simulink model "emg"  (R2014b)
settings: Solver=VariableStepAuto  StartTime=0.0  StopTime=10.0  RelTol=1e-3
libraries: simulink x1, instrumentlib x1, slrtlib x1
settings Model: Creator=Yue  LastModifiedBy=mLocal
settings DataIOCC: SaveFormat=Dataset
settings OptimizationCC: UseDivisionForNetSlopeComputation=off  SimCompilerOptimization=off
settings DebuggingCC: SolverPrmCheckMsg=none  FrameProcessingCompatibilityMsg=error  AllowSymbolicDim=off
settings HardwareCC: ProdBitPerPointer=64  ProdLargestAtomicFloat=Float  ProdIntDivRoundTo=Zero  ProdEndianess=LittleEndian  ProdHWDeviceType=Intel->x86-64 (Windows64)
settings RTWCC: RTWCompilerOptimization=off
settings GRTTargetCC: GeneratePreprocessorConditionals=Use local settings
settings ConfigComp: CovMetricSettings=dw  CovHtmlReporting=on  CovSaveCumulativeToWorkspaceVar=on  CovSaveSingleToWorkspaceVar=on  CovExternalEMLEnable=off

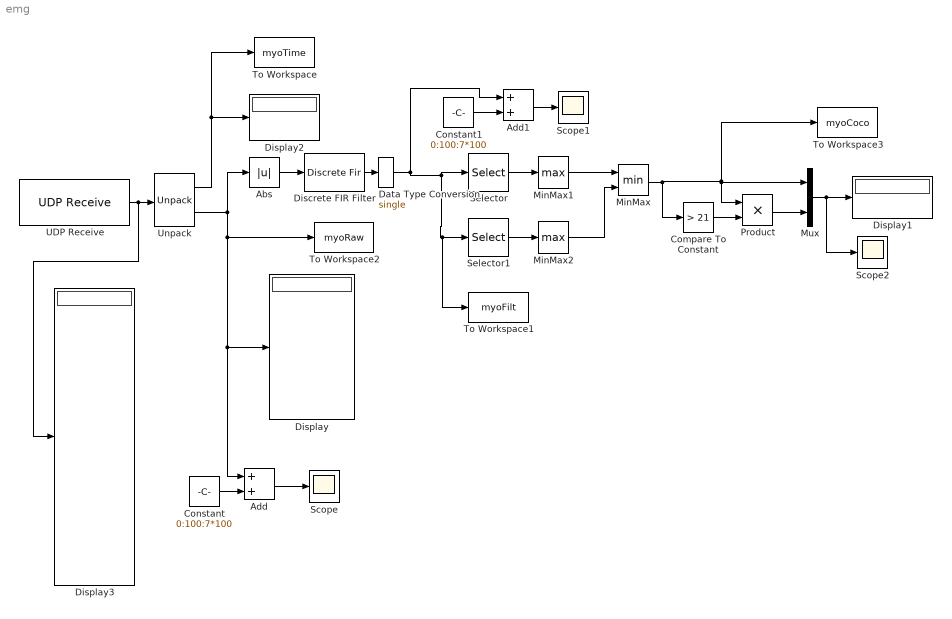
== system emg ==
  Abs : Abs
  Add : Sum
  Add1 : Sum
  Compare To Constant : simulink/Logic and Bit Operations/Compare To Constant  relop=>  const=21  OutDataTypeStr=uint8
  Constant : Constant  Value=0:100:7*100
  Constant1 : Constant  Value=0:100:7*100
  Data Type Conversion : DataTypeConversion  OutDataTypeStr=single
  Discrete FIR Filter : DiscreteFir  Coefficients=ones(1,100)/100
  Display{,1..3} (4 alike) : Display
  MinMax : MinMax  Inputs=2
  MinMax1 : MinMax  Function=max
  MinMax2 : MinMax  Function=max
  Mux : Mux  Inputs=2
  Product : Product
  Scope : Scope
      settings: ShowLegends=on  YMin=-100  YMax=800  MaxDataPoints=500000  SampleInput=on  SampleTime=0.005
  Scope1 : Scope
      settings: ShowLegends=on  YMin=0  YMax=800  MaxDataPoints=500000  SampleInput=on  SampleTime=0.005
  Scope2 : Scope
      settings: ShowLegends=on  TimeRange=19.93977176966292  YMin=0  YMax=100  SaveName=ScopeData2  MaxDataPoints=500000  SampleInput=on  SampleTime=0.005
  Selector : Selector  InputPortWidth=8  Indices=1:3
  Selector1 : Selector  InputPortWidth=8  Indices=6:8
  To Workspace : ToWorkspace  VariableName=myoTime  SaveFormat=Timeseries  SampleTime=-1
  To Workspace1 : ToWorkspace  VariableName=myoFilt  SaveFormat=Timeseries  SampleTime=-1
  To Workspace2 : ToWorkspace  VariableName=myoRaw  SaveFormat=Timeseries  SampleTime=-1
  To Workspace3 : ToWorkspace  VariableName=myoCoco  SaveFormat=Timeseries  SampleTime=-1
  UDP Receive : instrumentlib/UDP Receive  Host=127.0.0.1  Port=5689  LocalPort=8888  DataSize=16  EnableBlockingMode=on  Timeout=10  SampleTime=0.005  DataType=uint8  ByteOrder=BigEndian
  "Unpack " : slrtlib/UDP/Unpack   dimensions={[2],[8]}  datatypes={'uint32','int8'}  byteAlign=1
  wires:
  Add/1 -> Scope/1
  UDP Receive/1 -> Display3/1, "Unpack "/1
  Constant/1 -> Add/2
  Discrete FIR Filter/1 -> Data Type Conversion/1
  Add1/1 -> Scope1/1
  Constant1/1 -> Add1/2
  Selector/1 -> MinMax1/1
  Selector1/1 -> MinMax2/1
  Abs/1 -> Discrete FIR Filter/1
  Mux/1 -> Display1/1, Scope2/1
  Compare To Constant/1 -> Product/2
  MinMax1/1 -> MinMax/1
  MinMax2/1 -> MinMax/2
  MinMax/1 -> Compare To Constant/1, Product/1, Mux/1, To Workspace3/1
  Data Type Conversion/1 -> Add1/1, To Workspace1/1, Selector1/1, Selector/1
  "Unpack "/2 -> To Workspace2/1, Display/1, Add/1, Abs/1
  "Unpack "/1 -> To Workspace/1, Display2/1
  Product/1 -> Mux/2
